simulink model "Inductive_Balancing_Multiple_Cells"  (R2024b)
settings: Solver=VariableStepAuto  StartTime=0.0  StopTime=150  RelTol=1e-3
undefined symbols (not defined in the file): Ion, Lithium
libraries: spsIdealSwitchLib x10, spsDiodeLib x8, spsBatteryLib x4, spsSeriesRLCBranchLib x2, spsDCVoltageSourceLib x1, spsGroundLib x1, spsPWMGenerator2LevelLib x1, sps_lib x1
settings Model: Creator=yeswa  LastModifiedBy=yeswa

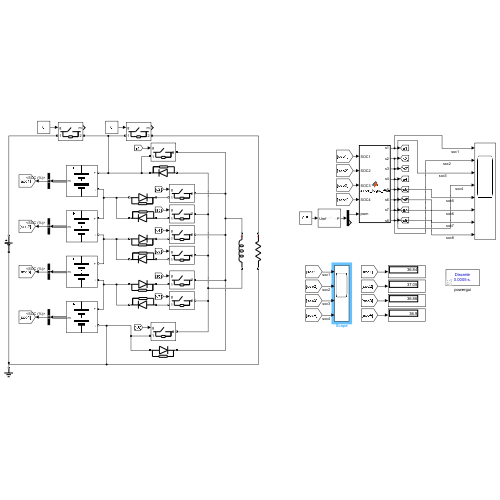
[thumbnail: Simulink's stored preview of the top-level diagram]
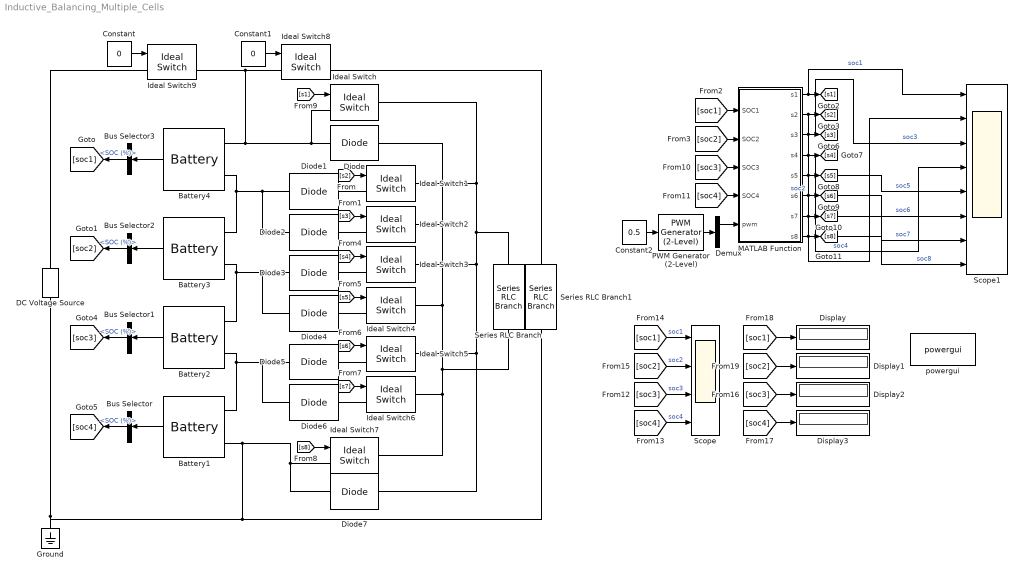
== system Inductive_Balancing_Multiple_Cells ==
  Battery1 : spsBatteryLib/Battery  BatType=Lithium-Ion  NomV=3.7  NomQ=5.4  SOC=32  Batt_Tr=30  PresetModel=on  MaxQ=5.4  MinV=2.775  FullV=4.3068  Dis_rate=2.3478  R=0.0068519  Normal_OP=4.8835  expZone="[3.9974      0.2653]"
  Battery2 : spsBatteryLib/Battery  BatType=Lithium-Ion  NomV=3.7  NomQ=5.4  SOC=45  Batt_Tr=30  PresetModel=on  MaxQ=5.4  MinV=2.775  FullV=4.3068  Dis_rate=2.3478  R=0.0068519  Normal_OP=4.8835  expZone="[3.9974      0.2653]"
  Battery3 : spsBatteryLib/Battery  BatType=Lithium-Ion  NomV=3.7  NomQ=5.4  SOC=35  Batt_Tr=30  PresetModel=on  MaxQ=5.4  MinV=2.775  FullV=4.3068  Dis_rate=2.3478  R=0.0068519  Normal_OP=4.8835  expZone="[3.9974      0.2653]"
  Battery4 : spsBatteryLib/Battery  BatType=Lithium-Ion  NomV=3.7  NomQ=5.4  SOC=40  Batt_Tr=30  PresetModel=on  MaxQ=5.4  MinV=2.775  FullV=4.3068  Dis_rate=2.3478  R=0.0068519  Normal_OP=4.8835  expZone="[3.9974      0.2653]"
  Bus Selector{,1..3} (4 alike) : BusSelector  OutputSignals=SOC (%)
  Constant : Constant  Value=0
  Constant1 : Constant  Value=0
  Constant2 : Constant  Value=0.5
  DC Voltage Source : spsDCVoltageSourceLib/DC Voltage Source  Amplitude=20  Measurements=None
  Demux : Demux  Outputs=2
  Diode{,1..7} (8 alike) : spsDiodeLib/Diode  Ron=0.001  Lon=0  Vf=0.8  IC=0  UseSnubber=0  Rs=500  Cs=250e-9  Measurements=off
  Display{,1..3} (4 alike) : Display
  Ground : spsGroundLib/Ground  LConnTagsString=a
  Ideal Switch{,1..7} (8 alike) : spsIdealSwitchLib/Ideal Switch  Ron=0.001  Lon=0  IC=0  Rs=1e5  Cs=inf  Measurements=off
  Ideal Switch8 : spsIdealSwitchLib/Ideal Switch  Ron=0.001  Lon=0  IC=0  Rs=1e5  Cs=inf  Measurements=on
  Ideal Switch9 : spsIdealSwitchLib/Ideal Switch  Ron=0.001  Lon=0  IC=0  Rs=1e5  Cs=inf  Measurements=on
  MATLAB Function : MATLAB Function  TreatAsAtomicUnit=on
  PWM Generator (2-Level) : spsPWMGenerator2LevelLib/PWM Generator (2-Level)  ModulatorType=Single-phase half-bridge (2 pulses)  ModulatorMode=Unsynchronized  Fc=500  Pc=0  nF=27  MinMax="[ -1  1 ]"  SamplingTechnique=Natural  ModulatingSignals=off  m=0.8  Freq=60  Phase=0  Ts=0  ShowCarrierOutport=off
  Scope : Scope  NumInputPorts=4
  Scope1 : Scope  NumInputPorts=8
  Series RLC Branch : spsSeriesRLCBranchLib/Series RLC Branch  LConnTagsString=__new0  RConnTagsString=__new0  BranchType=L  Resistance=1  Inductance=1e-3  SetiL0=off  InitialCurrent=0  Capacitance=1e-6  Setx0=off  InitialVoltage=0  Measurements=None
  Series RLC Branch1 : spsSeriesRLCBranchLib/Series RLC Branch  LConnTagsString=__new0  RConnTagsString=__new0  BranchType=R  Resistance=1  Inductance=1e-3  SetiL0=off  InitialCurrent=0  Capacitance=1e-6  Setx0=off  InitialVoltage=0  Measurements=None
  powergui : sps_lib/powergui  Priority=1  SimulationMode=Discrete  SampleTime=50e-5  frequency=60  Iterations=50  frequencyindice=0  Pbase=100e6  ErrMax=1e-4  UnitsV=kV  UnitsW=MW  buscounter=0  FunctionMessages=off  echomessages=off  EnableUseOfTLC=off  CurrentSourceSwitches=off  DisableSnubberDevices=off  DisableRonSwitches=off  DisableVfSwitches=off  DisplayEquations=off  AutomaticDiscreteSolvers=off  SolverType=Tustin/Backward Euler (TBE)  Interpol=off  ExternalGateDelay=off  methode=off  Ts=100  x0status=blocks  SPID=on  SwTol=0  HookPort=off  NonlinearTolerance=1e-4  nMaxIteration=100  ContinueOnMaxIteration=off  RestoreLinks=warning  ResistiveCurrentMeasurement=off  Frange=[0:2:500]  Ylog=off  Xlog=on  ShowGrid=off  save=off  variable=ZData  structure=0  ZoomFFT=off  StartTime=0.0  cycles=1  DisplayStyle=1  fundamental=60  FreqAxis=off  MaxFrequency=1000  frequencyindicesteady=1  RmsSteady=1  display=off
  wires:
  Battery1/1 -> Bus Selector/1
  Battery2/1 -> Bus Selector1/1
  Battery3/1 -> Bus Selector2/1
  Battery4/1 -> Bus Selector3/1
  Bus Selector3/1 -> [soc1]  "<SOC (%)>"
  Bus Selector2/1 -> [soc2]  "<SOC (%)>"
  Bus Selector1/1 -> [soc3]  "<SOC (%)>"
  Bus Selector/1 -> [soc4]  "<SOC (%)>"
  [s2] -> Ideal Switch1/1
  [s3] -> Ideal Switch2/1
  [s4] -> Ideal Switch3/1
  [s5] -> Ideal Switch4/1
  [s6] -> Ideal Switch5/1
  [s7] -> Ideal Switch6/1
  [s8] -> Ideal Switch7/1
  [s1] -> Ideal Switch/1
  Constant/1 -> Ideal Switch9/1
  Constant1/1 -> Ideal Switch8/1
  MATLAB Function/1(s1) -> Scope1/1, [s1]  "soc1"
  MATLAB Function/2(s2) -> Scope1/2, [s2]  "soc2"
  MATLAB Function/4(s4) -> Scope1/4, [s4]  "soc4"
  MATLAB Function/3(s3) -> Scope1/3, [s3]  "soc3"
  MATLAB Function/5(s5) -> Scope1/5, [s5]  "soc5"
  MATLAB Function/6(s6) -> Scope1/6, [s6]  "soc6"
  MATLAB Function/7(s7) -> Scope1/7, [s7]  "soc7"
  MATLAB Function/8(s8) -> Scope1/8, [s8]  "soc8"
  [soc1] -> MATLAB Function/1(SOC1)
  [soc2] -> MATLAB Function/2(SOC2)
  PWM Generator (2-Level)/1 -> Demux/1
  Constant2/1 -> PWM Generator (2-Level)/1
  Demux/1 -> MATLAB Function/5(pwm)
  [soc2] -> Scope/2  "soc2"
  [soc1] -> Scope/1  "soc1"
  [soc3] -> Scope/3  "soc3"
  [soc4] -> Scope/4  "soc4"
  [soc4] -> Display3/1
  [soc3] -> Display2/1
  [soc1] -> Display/1
  [soc2] -> Display1/1
  [soc3] -> MATLAB Function/3(SOC3)
  [soc4] -> MATLAB Function/4(SOC4)
  connections:
  Diode5/LConn1 -- Battery1/LConn1 -- Battery2/LConn2 -- Diode6/RConn1
  Diode4/RConn1 -- Battery3/LConn2 -- Battery2/LConn1 -- Diode3/LConn1
  Battery3/LConn1 -- Diode2/RConn1 -- Diode1/LConn1 -- Battery4/LConn2
  Ideal Switch1/LConn1 -- Diode1/RConn1
  Diode2/LConn1 -- Ideal Switch2/LConn1
  Diode4/LConn1 -- Ideal Switch4/LConn1
  Ideal Switch3/LConn1 -- Diode3/RConn1
  Ideal Switch5/LConn1 -- Diode5/RConn1
  Diode6/LConn1 -- Ideal Switch6/LConn1
  Ground/LConn1 -- Diode7/LConn1 -- Ideal Switch7/LConn1 -- Battery1/LConn2 -- Series RLC Branch1/RConn1 -- DC Voltage Source/LConn1
  Ideal Switch3/RConn1 -- Diode7/RConn1 -- Ideal Switch5/RConn1 -- Ideal Switch1/RConn1 -- Ideal Switch/RConn1 -- Series RLC Branch/LConn1
  Ideal Switch8/RConn1 -- Series RLC Branch1/LConn1
  Ideal Switch9/LConn1 -- DC Voltage Source/RConn1
  Ideal Switch7/RConn1 -- Series RLC Branch/RConn1 -- Ideal Switch4/RConn1 -- Ideal Switch2/RConn1 -- Diode/LConn1 -- Ideal Switch6/RConn1
  Diode/RConn1 -- Battery4/LConn1 -- Ideal Switch9/RConn1 -- Ideal Switch8/LConn1 -- Ideal Switch/LConn1

== matlab function Inductive_Balancing_Multiple_Cells/MATLAB Function ==
  settings: updateMethod=DISCRETE
  data: SOC1 input; s1 output; SOC2 input; SOC3 input; SOC4 input; pwm input; s2 output; s3 output; s4 output; s5 output; s6 output; s7 output; s8 output
function [s1, s2, s3, s4, s5, s6, s7, s8] = balance_logic_4cells(SOC1, SOC2, SOC3, SOC4, pwm)
% Inputs:
%   SOC1, SOC2, SOC3, SOC4 -> SOCs of cells (%)
%   pwm                     -> PWM input (0 or 1)
%
% Outputs:
%   s1-s8 -> switch control signals

% Persistent step counter
persistent stepCount
if isempty(stepCount)
    stepCount = int32(0);
end

% Initialize outputs
s1=0; s2=0; s3=0; s4=0; s5=0; s6=0; s7=0; s8=0;

% Threshold to avoid chatter
threshold = 0.5;

SOC = [SOC1, SOC2, SOC3, SOC4];

% Find highest and lowest SOC with threshold
[maxSOC, maxIdx] = max(SOC);
[minSOC, minIdx] = min(SOC);

if (maxSOC - minSOC) > threshold
    % Charging inductor from highest SOC when PWM=high
    if pwm == 1
        switch maxIdx
            case 1, s1 = 1; s3 = 1;
            case 2, s2 = 1; s5 = 1;
            case 3, s4 = 1; s7 = 1;
            case 4, s6 = 1; s8 = 1;
        end
    else
        % Discharging inductor to lowest SOC when PWM=low
        switch minIdx
            case 1, s2 = 1; % energy goes to cell1
            case 2, s3 = 1; s4 = 1; % energy goes to cell2
            case 3, s5 = 1; s6 = 1; % energy goes to cell3
            case 4, s7 = 1;  % energy goes to cell4
        end
    end
end

% Increment step counter
stepCount = stepCount + 1;

% Debug messages for first 500 steps
if stepCount <= 500
    fprintf('Step %d | SOC=[%.2f %.2f %.2f %.2f] | PWM=%d | s=[%d %d %d %d %d %d %d %d]\n', ...
        int32(stepCount), SOC1, SOC2, SOC3, SOC4, int32(pwm), ...
        int32(s1), int32(s2), int32(s3), int32(s4), int32(s5), int32(s6), int32(s7), int32(s8));
end

end
